simulink subsystem "MotoSimpleECU"  (R2024a)
settings: Solver=VariableStepAuto  StartTime=0.0  StopTime=10.0  RelTol=1e-3
undefined symbols (not defined in the file): CtrlEcuRevLim
settings Model: Creator=The MathWorks, Inc.  LastModifiedBy=The MathWorks, Inc.
settings RTWCC: GPUComputeCapability=3.5

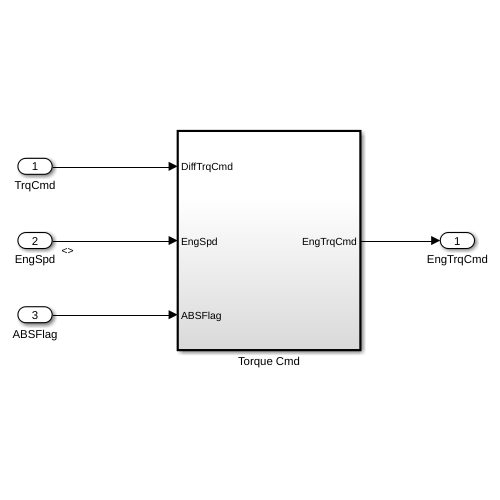
[thumbnail: Simulink's stored preview of the top-level diagram]
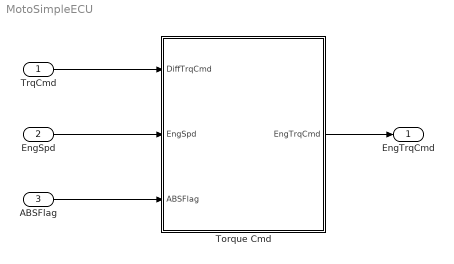
== system MotoSimpleECU ==
  TrqCmd : Inport
  EngSpd : Inport  Port=2
  ABSFlag : Inport  Port=3
  Torque Cmd : Subsystem  TreatAsAtomicUnit=on  SystemSampleTime=.01
  EngTrqCmd : Outport  VectorParamsAs1DForOutWhenUnconnected=off
  wires:
  ABSFlag/1 -> Torque Cmd/3(ABSFlag)
  Torque Cmd/1(EngTrqCmd) -> EngTrqCmd/1
  TrqCmd/1 -> Torque Cmd/1(DiffTrqCmd)
  EngSpd/1 -> Torque Cmd/2(EngSpd)

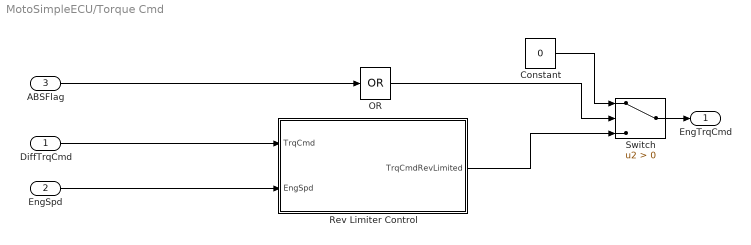
== system MotoSimpleECU/Torque Cmd ==
  DiffTrqCmd : Inport
  EngSpd : Inport  Port=2  Unit=rpm
  ABSFlag : Inport  Port=3
  Constant : Constant  Value=0
  OR : Logic  Operator=OR  Inputs=1  AllPortsSameDT=off  OutDataTypeStr=boolean
  Rev Limiter Control : Subsystem
  Switch : Switch  Criteria=u2 > Threshold  ZeroCross=off  SaturateOnIntegerOverflow=off  InputSameDT=off
  EngTrqCmd : Outport
  wires:
  DiffTrqCmd/1 -> Rev Limiter Control/1(TrqCmd)
  EngSpd/1 -> Rev Limiter Control/2(EngSpd)
  Rev Limiter Control/1(TrqCmdRevLimited) -> Switch/3
  Switch/1 -> EngTrqCmd/1
  ABSFlag/1 -> OR/1
  Constant/1 -> Switch/1
  OR/1 -> Switch/2

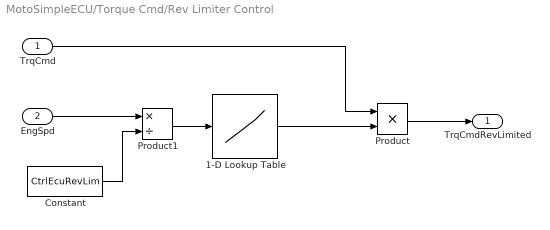
== system MotoSimpleECU/Torque Cmd/Rev Limiter Control ==
  TrqCmd : Inport
  EngSpd : Inport  Port=2
  1-D Lookup Table : Lookup_n-D  NumberOfTableDimensions=1  BreakpointsForDimension1=[1 1.01]  Table=[1 0]  ExtrapMethod=Clip  InternalRulePriority=Speed  RndMeth=Simplest
  Constant : Constant  Value=CtrlEcuRevLim
  Product : Product
  Product1 : Product  Inputs=*/
  TrqCmdRevLimited : Outport  VectorParamsAs1DForOutWhenUnconnected=off
  wires:
  EngSpd/1 -> Product1/1
  Product/1 -> TrqCmdRevLimited/1
  1-D Lookup Table/1 -> Product/2
  TrqCmd/1 -> Product/1
  Constant/1 -> Product1/2
  Product1/1 -> 1-D Lookup Table/1
